simulink model "sim_Motor_2kW_openloop_v2"
settings: Solver=ode45  StartTime=0.0  StopTime=0.03  RelTol=1e-3
libraries: powerlib x18
settings Model: Creator=Kun Zhang  LastModifiedBy=LYN
settings SolverCC: AutoInsertRateTranBlk=on
settings DataIOCC: LimitDataPoints=on  SaveFormat=Array  SignalLoggingSaveFormat=ModelDataLogs  ReturnWorkspaceOutputs=off
settings OptimizationCC: ExpressionDepthLimit=2147483647  LifeSpan=inf  SimCompilerOptimization=Off
settings DebuggingCC: UnderspecifiedInitializationDetection=Classic  MergeDetectMultiDrivingBlocksExec=none  SolverPrmCheckMsg=warning  MultiTaskDSMMsg=warning  MultiTaskCondExecSysMsg=none  FcnCallInpInsideContextMsg=Enable All  FrameProcessingCompatibilityMsg=warning  StateNameClashWarn=warning  StrictBusMsg=None  SFUnexpectedBacktrackingDiag=warning  SFNoUnconditionalDefaultTransitionDiag=warning
settings HardwareCC: ProdBitPerPointer=32  ProdLargestAtomicFloat=None  ProdIntDivRoundTo=Undefined  ProdEndianess=Unspecified  ProdWordSize=32  ProdHWDeviceType=32-bit Generic
settings ModelReferenceCC: PropagateSignalLabelsOutOfModel=off
settings SFSimCC: SimUseLocalCustomCode=off
settings RTWCC: RTWUseLocalCustomCode=off  IncludeERTFirstTime=on  RTWCompilerOptimization=Off
settings CodeAppCC: CustomSymbolStrType=$N$R$M
settings GRTTargetCC: CodeReplacementLibrary=ANSI_C  GeneratePreprocessorConditionals=Disable all  CombineOutputUpdateFcns=off  CPPClassGenCompliant=off  GRTInterface=on

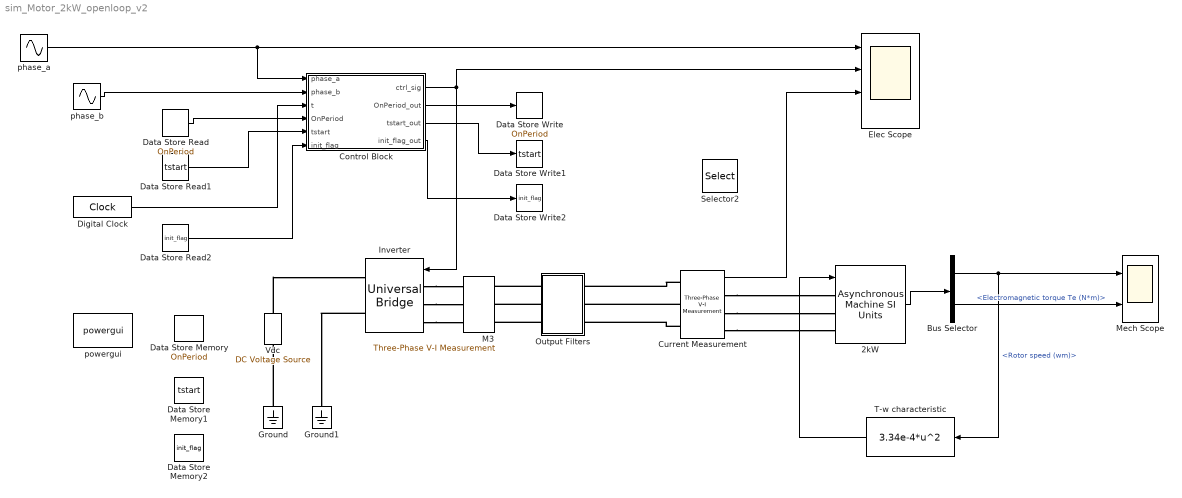
== system sim_Motor_2kW_openloop_v2 ==
  2kW : powerlib/Machines/Asynchronous Machine SI Units  PresetModel=No  MechanicalLoad=Torque Tm  ShowDetailedParameters=on  RotorType=Squirrel-cage  ReferenceFrame=Rotor  NominalParameters=[ 2000, 220, 50 ]  Stator=[ 1.115 0.005974]  Rotor=[ 1.083 0.005974]  Cage1=[ 0.022 0.226/377]  Cage2=[ 0.022 0.226/377]  Lm=0.2037  Mechanical=[0.02 0.005752 2]  PolePairs=2  InitialConditions=[1 0 0 0 0 0 0 0]  Units=SI  LoadFlowParameters=1492000  SimulateSaturation=off  Saturation=[14.03593122, 27.81365428, 53.79336849, 72.68890987, 97.98006896, 148.6815601, 215.7428561, 302.9841135, 428.7778367 ; 230, 322, 414, 460, 506, 552, 598, 644, 690]  TsPowergui=0  TsBlock=-1  IterativeModel=Forward Euler  Pmec=0
  Bus Selector : BusSelector  OutputSignals=Mechanical.Rotor speed (wm),Mechanical.Electromagnetic torque Te (N*m)
  Control Block : MATLAB Function  TreatAsAtomicUnit=on
  Current Measurement : powerlib/Measurements/Three-Phase V-I Measurement  VoltageMeasurement=no  SetLabelV=off  LabelV=Vabc  Vpu=off  VpuLL=off  CurrentMeasurement=yes  SetLabelI=off  LabelI=Iabc  Ipu=off  Pbase=100e6  Vbase=500e3  OutputType=Complex  PhasorSimulation=off  PSBequivalent=0
  Data Store Memory : DataStoreMemory  DataStoreName=OnPeriod  ReadBeforeWriteMsg=warning  WriteAfterWriteMsg=warning  WriteAfterReadMsg=warning
  Data Store Memory1 : DataStoreMemory  DataStoreName=tstart  ReadBeforeWriteMsg=warning  WriteAfterWriteMsg=warning  WriteAfterReadMsg=warning
  Data Store Memory2 : DataStoreMemory  DataStoreName=init_flag  ReadBeforeWriteMsg=warning  WriteAfterWriteMsg=warning  WriteAfterReadMsg=warning  OutMin=0  OutMax=1
  Data Store Read : DataStoreRead  DataStoreName=OnPeriod  DataStoreElements=OnPeriod
  Data Store Read1 : DataStoreRead  DataStoreName=tstart
  Data Store Read2 : DataStoreRead  DataStoreName=init_flag  DataStoreElements=init_flag
  Data Store Write : DataStoreWrite  DataStoreName=OnPeriod  DataStoreElements=OnPeriod
  Data Store Write1 : DataStoreWrite  DataStoreName=tstart  DataStoreElements=tstart
  Data Store Write2 : DataStoreWrite  DataStoreName=init_flag  DataStoreElements=init_flag
  Digital Clock : DigitalClock  SampleTime=1/(100*1000)
  "Elec Scope " : Scope  NumInputPorts=4
      settings: TimeRange=0.01  YMin=-1~0~-100~-1  YMax=1~2~125~1  SaveName=motor_2kW_elec
  Ground : powerlib/Elements/Ground  LConnTagsString=a
  Ground1 : powerlib/Elements/Ground  LConnTagsString=a
  Inverter : powerlib/Power Electronics/Universal Bridge  Arms=3  SnubberResistance=5000  SnubberCapacitance=inf  Device=IGBT / Diodes  Ron=1e-3  Lon=0  ForwardVoltages="[  0  0  ]"  ForwardVoltage=0  GTOparameters=[ 10e-6 , 20e-6 ]  IGBTparameters=[ 1e-6 , 1e-6 ]  Measurements=None  Measurements_2=None  converterType=Rectifier
  M3 : powerlib/Measurements/Three-Phase V-I Measurement  VoltageMeasurement=phase-to-ground  SetLabelV=on  LabelV=Vabc_M3  Vpu=off  VpuLL=off  CurrentMeasurement=yes  SetLabelI=on  LabelI=Iabc_M3  Ipu=off  Pbase=100e6  Vbase=500e3  OutputType=Complex  PhasorSimulation=off  PSBequivalent=0
  Mech Scope : Scope  NumInputPorts=2
      settings: TimeRange=0.01  YMin=-1~-5  YMax=1~5  SaveName=motor_2kW_mech
  Output Filters : Subsystem
  Selector2 : Selector  InputPortWidth=6  IndexOptions=Index vector (dialog)  Indices=[1]  OutputSizes=1
  T-w characteristic : Fcn  Expr=3.34e-4*u^2
  Vdc : powerlib/Electrical Sources/DC Voltage Source  Amplitude=400  Measurements=None
  "phase_a " : Sin  Frequency=2*pi*300  SampleTime=1/(100*1000)
  "phase_b " : Sin  Frequency=2*pi*300  Phase=2*pi/3  SampleTime=1/(100*1000)
  powergui : powerlib/powergui  Priority=1  SimulationMode=Discrete  SolverType=Tustin  SampleTime=10e-6  frequency=60  SPID=off  DisableSnubberDevices=off  DisableRonSwitches=off  DisableVfSwitches=off  SwTol=0  Interpol=off  DisplayEquations=off  FunctionMessages=off  frequencyindice=50  Pbase=100e6  ErrMax=1e-4  Iterations=50  UnitsV=kV  UnitsW=MW  echomessages=off  HookPort=off  EnableUseOfTLC=off  x0status=blocks  RestoreLinks=warning  ResistiveCurrentMeasurement=off  Ylog=off  Xlog=on  ShowGrid=off  save=off  variable=ZData  structure=motor_2kW_elec  ZoomFFT=off  StartTime=0.0  cycles=1  DisplayStyle=1  fundamental=60  FreqAxis=off  MaxFrequency=1000  frequencyindicesteady=1  display=off  methode=off
  wires:
  2kW/1 -> Bus Selector/1
  Bus Selector/1 -> T-w characteristic/1, Mech Scope/1  "<Rotor speed (wm)>"
  Bus Selector/2 -> Mech Scope/2  "<Electromagnetic torque Te (N*m)>"
  T-w characteristic/1 -> 2kW/1
  "phase_b "/1 -> Control Block/2(phase_b)
  Control Block/1(ctrl_sig) -> Inverter/1, "Elec Scope "/2
  Digital Clock/1 -> Control Block/3(t)
  "phase_a "/1 -> Control Block/1(phase_a), "Elec Scope "/1
  Data Store Read/1 -> Control Block/4(OnPeriod)
  Control Block/2(OnPeriod_out) -> Data Store Write/1
  Data Store Read1/1 -> Control Block/5(tstart)
  Control Block/3(tstart_out) -> Data Store Write1/1
  Data Store Read2/1 -> Control Block/6(init_flag)
  Control Block/4(init_flag_out) -> Data Store Write2/1
  Current Measurement/1 -> "Elec Scope "/3
  connections:
  Ground/LConn1 -- Vdc/LConn1
  Vdc/RConn1 -- Inverter/RConn1
  Inverter/RConn2 -- Ground1/LConn1
  Inverter/LConn1 -- M3/LConn1
  Inverter/LConn2 -- M3/LConn2
  Inverter/LConn3 -- M3/LConn3
  Output Filters/LConn1 -- M3/RConn1
  Output Filters/LConn2 -- M3/RConn2
  Output Filters/LConn3 -- M3/RConn3
  Current Measurement/RConn1 -- 2kW/LConn1
  Current Measurement/RConn2 -- 2kW/LConn2
  Current Measurement/RConn3 -- 2kW/LConn3
  Current Measurement/LConn1 -- Output Filters/RConn1
  Current Measurement/LConn2 -- Output Filters/RConn2
  Current Measurement/LConn3 -- Output Filters/RConn3

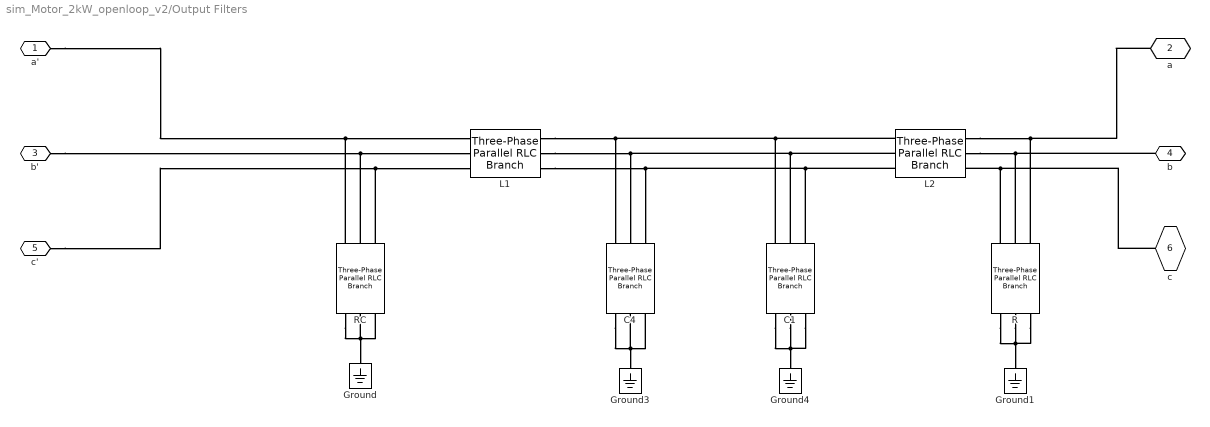
== system sim_Motor_2kW_openloop_v2/Output Filters ==
  C1 : powerlib/Elements/Three-Phase Parallel RLC Branch  LConnTagsString=A|B|C  RConnTagsString=A|B|C  BranchType=C  Resistance=1.5e6  Inductance=0.15e-5  Capacitance=10e-9  Measurements=None
  C4 : powerlib/Elements/Three-Phase Parallel RLC Branch  LConnTagsString=A|B|C  RConnTagsString=A|B|C  BranchType=C  Resistance=1.5e6  Inductance=0.15e-5  Capacitance=22e-6  Measurements=None
  Ground{,1,3..4} (4 alike) : powerlib/Elements/Ground  LConnTagsString=a
  L1 : powerlib/Elements/Three-Phase Parallel RLC Branch  LConnTagsString=A|B|C  RConnTagsString=A|B|C  BranchType=L  Resistance=1  Inductance=0.7e-1  Capacitance=1e-6  Measurements=None
  L2 : powerlib/Elements/Three-Phase Parallel RLC Branch  LConnTagsString=A|B|C  RConnTagsString=A|B|C  BranchType=L  Resistance=1  Inductance=1.4e-3  Capacitance=1e-6  Measurements=None
  "R " : powerlib/Elements/Three-Phase Parallel RLC Branch  LConnTagsString=A|B|C  RConnTagsString=A|B|C  BranchType=R  Resistance=100  Inductance=0.15e-5  Capacitance=20e-9  Measurements=None
  RC : powerlib/Elements/Three-Phase Parallel RLC Branch  LConnTagsString=A|B|C  RConnTagsString=A|B|C  BranchType=RC  Resistance=1.5e6  Inductance=0.15e-5  Capacitance=22e-6  Measurements=None
  " a'" : PMIOPort  Port=1  Side=Left
  a : PMIOPort  Port=2  Side=Right
  b' : PMIOPort  Port=3  Side=Left
  b : PMIOPort  Port=4  Side=Right
  c' : PMIOPort  Port=5  Side=Left
  c : PMIOPort  Port=6  Side=Right
  connections:
  RC/RConn1 -- " a'"/RConn1 -- L1/LConn1
  RC/RConn2 -- b'/RConn1 -- L1/LConn2
  RC/RConn3 -- c'/RConn1 -- L1/LConn3
  RC/LConn3 -- RC/LConn1 -- Ground/LConn1 -- RC/LConn2
  "R "/RConn2 -- L2/RConn2 -- b/RConn1
  "R "/LConn1 -- "R "/LConn3 -- "R "/LConn2 -- Ground1/LConn1
  L1/RConn1 -- L2/LConn1 -- C1/RConn1 -- C4/RConn1
  L1/RConn2 -- C1/RConn2 -- L2/LConn2 -- C4/RConn2
  L1/RConn3 -- C1/RConn3 -- L2/LConn3 -- C4/RConn3
  a/RConn1 -- L2/RConn1 -- "R "/RConn3
  c/RConn1 -- "R "/RConn1 -- L2/RConn3
  C4/LConn2 -- Ground3/LConn1 -- C4/LConn1 -- C4/LConn3
  C1/LConn3 -- C1/LConn1 -- Ground4/LConn1 -- C1/LConn2

== matlab function sim_Motor_2kW_openloop_v2/Control Block ==
  data: phase_a input; ctrl_sig output; phase_b input; t input; OnPeriod_out output; OnPeriod input; tstart input; tstart_out output; init_flag input; init_flag_out output
function	[ctrl_sig,OnPeriod_out,tstart_out,init_flag_out]= ctrl_blk_v2(phase_a,phase_b,t,OnPeriod,tstart,init_flag)
%%%%%%%%%%%%%%%%%%%%%%%%%%%%%%%%%%%%%%%%%%%%%%%%%%%%%%%%%%%%%%%%%%%%%%%%%%%%%%%%%%%%%%%%%%%%%%%%%%%%%%%%%%%%%%%%%%%%%%%%%%%%%%%%%%%%%%%%%%%%%%%%%%%%%%%%%%%%%%%%%
%                                                                                                                                                               %
%           The aim is to:                                                                                                                                      %                                                           
%           generate 3-phase PWM waveform using principle of PWM in simulink                                                                                    %                      
%           Version 1, written by Kun Zhang                                                                                                                     %                                          
%                                                                                                                                                               %
%           The input parameters are                                                                                                                            %                                               
%           phase_a: reference signal a                                                                                                                         %                              
%           phase_b: reference signal b                                                                                                                         %         
%           t: running time                                                                                                                                     %                      
%           fb_phase_a: feedback signal a                                                                                                                       %                                             
%           fb_phase_a: feedback signal b                                                                                                                       %
%           ton: on period                                                                                                                                      %
%           tstart: start time                                                                                                                                  %
%           init_flag:initial flag used to record the first tstart                                                                                              %
%                                                                                                                                                               %
%%%%%%%%%%%%%%%%%%%%%%%%%%%%%%%%%%%%%%%%%%%%%%%%%%%%%%%%%%%%%%%%%%%%%%%%%%%%%%%%%%%%%%%%%%%%%%%%%%%%%%%%%%%%%%%%%%%%%%%%%%%%%%%%%%%%%%%%%%%%%%%%%%%%%%%%%%%%%%%%%
%space reserved for gloabal variables declaration


%%%%%%%%%%%%%%%%%%%%%%%%%%%%%%%%%%%%%%%%%%%%%%%%%%%%%%%%%%%%%%%%%%%%%%%%%%%%%%%%%%%%%%%%%%%%%%%%%%%%%%%%%%%%%%%%%%%%%%%%%%%%%%%%%%%%%%%%%%%%%%%%%%%%%%%%%%%%%%%%%
REF_AMP= 1;                                                                 %magnitude of reference
REC_FREQ= 1500;                                                             %frequency of PWM 
REC_PER= 1/REC_FREQ;                                                        %period of PWM 
VON= REF_AMP*2;                                                             %set on voltage =2* reference voltage


%%%%%%%%%%%%%%%%%%%%%%%%%%%%%%%%%%%%%%%%%%%%%%%%%%%%%%%%%%%%%%%%%%%%%%%%%%%%%%%%%%%%%%%%%%%%%%%%%%%%%%%%%%%%%%%%%%%%%%%%%%%%%%%%%%%%%%%%%%%%%%%%%%%%%%%%%%%%%%%%%
phase_a= phase_a+REF_AMP;                                                   %shift phase_a by REF_AMP
phase_b= phase_b+REF_AMP;                                                   %shift phase_b by REF_AMP
phase_c= -phase_a-phase_b;                                                  %phase_c obatined by phase_a and phase_b


%%%%%%%%%%%%%%%%%%%%%%%%%%%%%%%%%%%%%%%%%%%%%%%%%%%%%%%%%%%%%%%%%%%%%%%%%%%%%%%%%%%%%%%%%%%%%%%%%%%%%%%%%%%%%%%%%%%%%%%%%%%%%%%%%%%%%%%%%%%%%%%%%%%%%%%%%%%%%%%%%
%when t less than one rectangular period
InitialTime= tstart+REC_PER;                                                %initial setting up time
D_a= phase_a/VON;                                                           %duty cycle for phase a
OnPeriod= D_a*REC_PER;                                                      %on period for a block
OffTime= tstart+OnPeriod;                                                   %the block is on unitl OffTime

if      t<InitialTime;
        if      init_flag==0
                t= tstart;              init_flag= 1;
        end
        if      t<=OffTime;           	pwm_1= VON;                
        else    pwm_1= 0;
        end
end

%when t greater than 1 rectangular period
if      t>InitialTime;
        tstart= t;                                                          %record the start time
        pwm_1= 1;                                                           %initial value of pwm_1 is set to 1
        elseif      t<=OffTime;              pwm_1= VON;           
        else        pwm_1= 0;
end

% Delay
%pause on;                pause(1*10^-6);                pause off;         %pausing for switching time (typically less than 1us)
if      pwm_1==0;                       pwm_2= VON;
else                                    pwm_2= 0;
end

% if      pwm_3==0;                       pwm_4= VON;
% else    pwm_4= 0;
% end
% 
% if      pwm_5==0;                       pwm_6= VON;
% else    pwm_6= 0;
% end


% 
% if t>tstart+REC_PER;
%             D= phase_b/VON;                     %duty cycle for phase b
%             tstart= t;                          %record the start time
%             ton= D*REC_PER;                     %on time
% elseif t<=(tstart+ton)
%                         pwm_3= VON;             %pwm3 on               
%                         pwm_4= 0;               %pwm4 off
%     else
%                         pwm_3= VON;             %pwm3 on               
%                         pwm_4= 0;               %pwm4 off
% end
% 
% if t>tstart+REC_PER;
%             D= phase_c/VON;                     %duty cycle for phase a
%             tstart= t;                          %record the start time
%             ton= D*REC_PER;                     %on time
% elseif t<=(tstart+ton)
%                         pwm_5= VON;             %pwm5 on               
%                         pwm_6= 0;               %pwm6 off
%     else
%                         pwm_5= VON;             %pwm5 on               
%                         pwm_6= 0;               %pwm6 off
% end

%PWM3~PWM6 temporarily assign to zero
pwm_3= 0;
pwm_4= 0;
pwm_5= 0;
pwm_6= 0;


%%%%%%%%%%%%%%%%%%%%%%%%%%%%%%%%%%%%%%%%%%%%%%%%%%%%%%%%%%%%%%%%%%%%%%%%%%%%%%%%%%%%%%%%%%%%%%%%%%%%%%%%%%%%%%%%%%%%%%%%%%%%%%%%%%%%%%%%%%%%%%%%%%%%%%%%%%%%%%%%%
OnPeriod_out= OnPeriod;                                                     %save ton in memeory
tstart_out= tstart;                                                         %save tstart in memeory
init_flag_out= init_flag;                                                   %save init_flag in memory
ctrl_sig= [pwm_1 pwm_2 pwm_3 pwm_4 pwm_5 pwm_6];                            %six phase PWM
